simulink model "TechnoEconomicMicrogrid"  (R2025a)
settings: Solver=VariableStepAuto  StartTime=0.0  StopTime=tPeriod-1  FixedStep=sampleTime  RelTol=1e-3
PostLoadFcn:
  | TechnoEconomicAnalysisInput
undefined symbols (not defined in the file): batteryProfile, batteryStorage, DiscIntNeverNeededParam, EMS, generatorProfile, generatorSet, line, loadForecast, mainGrid, optimizationInterval, optimizationMode, solarForecast, solarPV, windFarm, windForecast, windPowerEst
libraries: ee_lib x11, fl_lib x9, simulink x5, eeGeneralControl x4, nesl_utility x3, simulink_extras x1
(part 1 of 2)
CloseFcn:
  | figure1 = findobj('Type', 'figure', 'Name','Power Flow in Microgrid');
  | figure2 = findobj('Type', 'figure', 'Name','plot_PowerFlow');
  | figure3 = findobj('Type', 'figure', 'Name','plot_costComparison');
  | figure4 = findobj('Type', 'figure', 'Name','plot_totalCost');
  | figure5 = findobj('Type', 'figure', 'Name','plot_powerInRange');
  | 
  | if ~isempty(figure1)
  |     close(figure1);
  | end
  | if ~isempty(figure2)
  |     close(figure2);
  | end
  | if ~isempty(figure3)
  |     close(figure3);
  | end
  | if ~isempty(figure4)
  |     close(figure4);
  | end
  | if ~isempty(figure5)
  |     close(figure5);
  | end
  | clear figure1 figure2 figure3 figure4 figure5
  | if bdIsLoaded('SolarMPPTTestHarness')
  |     try
  |         close_system('SolarMPPTTestHarness');
  |     catch
  |     end
  | end
  | if bdIsLoaded('WindMPPTTestHarness')
  |       try
  |         close_system('WindMPPTTestHarness');
  |         catch
  |       end
  | end
settings Model: SimulationMode=accelerator  Creator=skota  LastModifiedBy=skota
settings DataIOCC: SaveOutput=off  DSMLogging=off  SaveTime=off  OutputSaveName=logsout
settings DebuggingCC: SFUnusedDataAndEventsDiag=none
settings ModelReferenceCC: PropagateVarSize=During execution

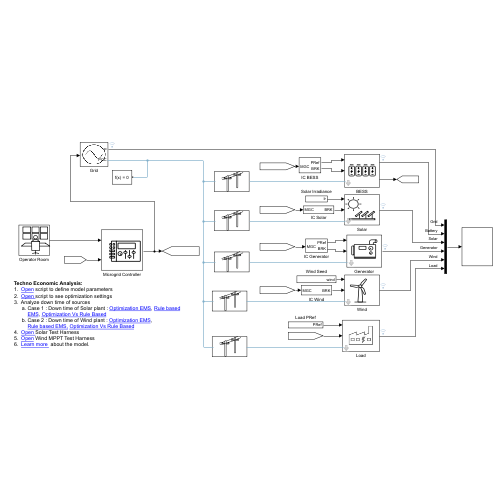
[thumbnail: Simulink's stored preview of the top-level diagram]
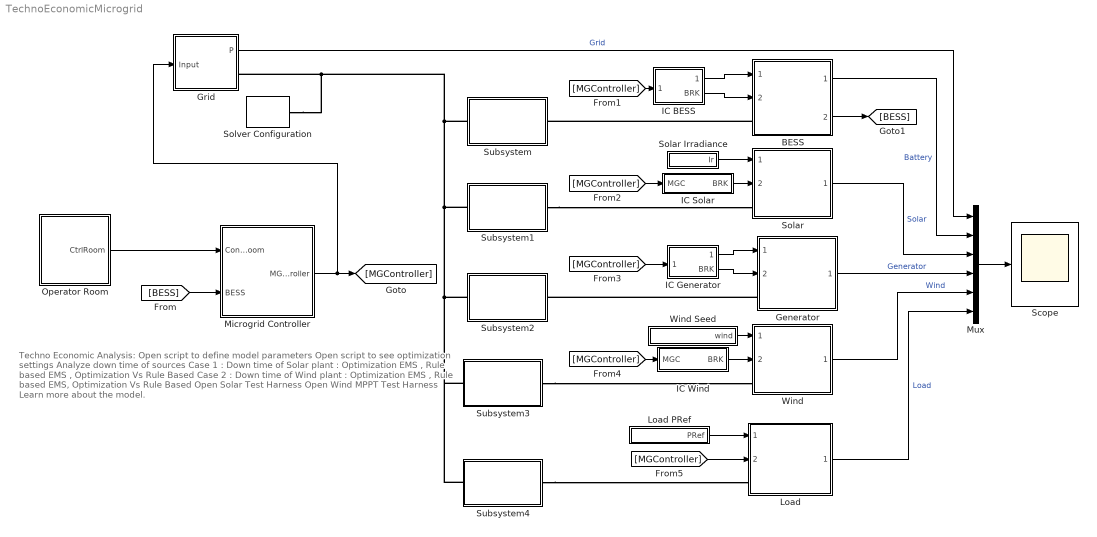
== system TechnoEconomicMicrogrid ==
  note: Techno Economic Analysis:
      | Open script to define model parameters
      | Open script to see optimization settings
      | Analyze down time of sources
      | Case 1 : Down time of Solar plant : Optimization EMS , Rule based EMS , Optimization Vs Rule Based
      | Case 2 : Down time of Wind plant : Optimization EMS ,
      | Rule based EMS, Optimization Vs Rule Based
      | Open Solar Test Harness
      | Open Wind MPPT Test Harness
      | Learn more about the model.
  BESS : Subsystem  ReferencedSubsystem=Battery  minSOC=batteryStorage.minSOC  maxSOC=batteryStorage.maxSOC  energyRating=batteryStorage.energyRating  capacityRating=batteryStorage.capacityRating  nominalVoltage=batteryStorage.nominalVoltage  frequency=systemFrequency  windingRatio=batteryStorage.windingRatio
  Generator : Subsystem  ReferencedSubsystem=Generator  genRating=generatorSet.rating  ratedVoltage=690%generatorSet.voltage  ratedFrequency=systemFrequency  polePairs=generatorSet.polePairs  windingRatio=generatorSet.transformerRatio
  Grid : Subsystem
      settings: PortSchema="{\"entries\":[{\"content\":{\"sides\":[{\"content\":{},\"type\":\"ConnectorPlacement.EquallySpacedRectSide\",\"uuid\":\"0399238b-9a5e-45cc-8714-91426baf51ba\"},{\"content\":{\"side\":\"RIGHT\"},\"type\":\"ConnectorPlacement.EquallySpacedRectSide\",\"uuid\":\"f3b9b3de-730a-435e-bd02-72046c7f84f4\"},{\"content\":{\"connectorIds\":[\"In1\"],\"side\":\"TOP\"},\"type\":\"ConnectorPlacement.EquallySpacedRectSide\",\"uuid\":\"aa72cc88-43a3-4304-9895-61739a7354ea\"},{\"content\":{\"connectorIds\":[\"Out1\",\"RConn1\"],\"side\":\"BOTTOM\"},\"type\":\"ConnectorPlacement.EquallySpacedRectSide\",\"uuid\":\"4abd50ca-018b-43d1-adba-697df11ba2b3\"}]},\"type\":\"ConnectorPlacement.EquallySpacedConnector\",\"uuid\":\"8478d8ff-3240-4ebb-965c-af7f48cfdc7b\"}],\"packageUris\":[\"http://schema.mathworks.com/mf0/Connector/R2020b\"],\"version\":\"1.0\"}"
      mask Display: image('Maingrid.svg');
  IC BESS : Subsystem
  IC Generator : Subsystem
  IC Solar : Subsystem
  IC Wind : Subsystem
  Load : Subsystem  ReferencedSubsystem=Load  windingRatio=loadParam.transformerRatio
  Load PRef : Subsystem
  Microgrid Controller : Subsystem
  Mux : Mux  Inputs=6
  Operator Room : Subsystem
  Scope : Scope
      settings: ActiveDisplayYMinimum=-294.67014  ActiveDisplayYMaximum=1651.08845
  Solar : Subsystem  ReferencedSubsystem=Solar  maxSolarIrradiance=solarPV.maxIrradiance  solarRating=solarPV.rating  ratedVoltage=solarPV.voltage  Voc=solarPV.Voc  panelOutput=solarPV.panelOutput  frequency=systemFrequency  windingRatio=solarPV.transformerRatio  MPPTVoltage=solarMPPT.vMPP  MPPTIrradiance=solarMPPT.irradiance
  Solar Irradiance : Subsystem
  Solver Configuration : nesl_utility/Solver Configuration  PhysicalDomain=network_engine_domain  SubClassName=solver  LeftPortType=input  RightPortType=generic  Tones=[]  Harmonics=[]  SimulateNoise=off  Profile=off  UseLocalSampling=off  EnableSwitchedLinearOptims=on  FrequencyDomain=off  UseCCode=off  RelTol=0.001  AbsTol=0.001  MinStep=1e-09  ToWorkspace=off  RevertToSquareIcSolve=off  NumHomotopyIterations=100  PhasorMode=off  PhasorModeNumHarmonics=1  ConsistencySolver=NEWTON_XTOL_AFTER_FTOL  IndexReductionMethod=DerivativeReplacement  DoDC=off  ResidualTolerance=1e-09  ConsistencyTolSource=GLOBAL  ConsistencyAbsTol=0.001  ConsistencyRelTol=0.001  ConsistencyTolFactor=1  UseLocalSolver=on  LocalSolverChoice=NE_BACKWARD_EULER_ADVANCER  ResolveIndetEquations=on  FunctionEvalNumThread=1  LocalSolverSampleTime=sampleTime  DoFixedCost=on  MaxNonlinIter=3  MaxModeIter=2  ComputeImpulses=off  ImpulseIterations=2  LinearAlgebra=Sparse  LinearAlgebraNumThread=0  EquationFormulation=NE_FREQUENCY_TIME_EF  DelaysMemoryBudget=1024  AutomaticFiltering=on  FilteringTimeConstant=0.001  PartitionStorageMethod=AS_NEEDED  PartitionMemoryBudget=1024  PartitionMethod=ROBUST  MultibodyUseLocalSolver=off  MultibodyLocalSolverChoice=ODE1  MultibodyLocalSolverSampleTime=0.001
  Subsystem : Subsystem
  Subsystem1 : Subsystem
  Subsystem2 : Subsystem
  Subsystem3 : Subsystem
  Subsystem4 : Subsystem
  Wind : Subsystem  ReferencedSubsystem=Wind  windRating=windFarm.rating  maxWindSpeed=windFarm.maxWindSpeed  turbineOutput=windFarm.turbineOutput  frequency=systemFrequency  windingRatio=windFarm.transformerRatio  rotorSpeed=windMPPT.rotorSpeed  windSpeed=windMPPT.windSpeed
  Wind Seed : Subsystem
  wires:
  Grid/1(P) -> Mux/1  "Grid"
  BESS/1 -> Mux/2  "Battery"
  Solar/1 -> Mux/3  "Solar"
  Generator/1 -> Mux/4  "Generator"
  Wind/1 -> Mux/5  "Wind"
  Load/1 -> Mux/6  "Load"
  Operator Room/1(CtrlRoom) -> Microgrid Controller/1(Control Room)
  Microgrid Controller/1(MGController) -> Grid/1(Input), [MGController]
  [BESS] -> Microgrid Controller/2(BESS)
  [MGController] -> IC Wind/1(MGC)
  [MGController] -> Load/2
  Mux/1 -> Scope/1
  BESS/2 -> [BESS]
  [MGController] -> IC BESS/1(MGC)
  IC BESS/2(BRK) -> BESS/2
  IC BESS/1(PRef) -> BESS/1
  [MGController] -> IC Solar/1(MGC)
  IC Solar/1(BRK) -> Solar/2
  IC Wind/1(BRK) -> Wind/2
  Solar Irradiance/1(Ir) -> Solar/1
  IC Generator/1(PRef) -> Generator/1
  Wind Seed/1(wind) -> Wind/1
  Load PRef/1(PRef) -> Load/1
  [MGController] -> IC Generator/1(MGC)
  IC Generator/2(BRK) -> Generator/2
  connections:
  Subsystem4/LConn1 -- Subsystem3/LConn1 -- Subsystem1/LConn1 -- Subsystem/LConn1 -- Solver Configuration/RConn1 -- Grid/RConn1 -- Subsystem2/LConn1
  BESS/LConn1 -- Subsystem/RConn1
  Subsystem1/RConn1 -- Solar/LConn1
  Generator/LConn1 -- Subsystem2/RConn1
  Subsystem3/RConn1 -- Wind/LConn1
  Subsystem4/RConn1 -- Load/LConn1

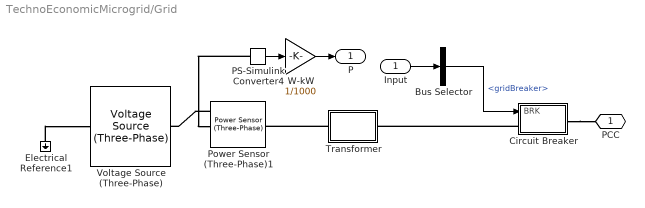
== system TechnoEconomicMicrogrid/Grid ==
  Input : Inport
  Bus Selector : BusSelector  OutputSignals=BrkControl.gridBreaker
  Circuit Breaker : Subsystem
  Electrical Reference1 : fl_lib/Electrical/Electrical Elements/Electrical Reference
  PS-Simulink Converter4 : nesl_utility/PS-Simulink Converter  PhysicalDomain=network_engine_domain  SubClassName=ps_output  LeftPortType=input  RightPortType=output  PseudoPeriodic=off  Frequencies=[]  VectorFormat=inherit  Unit=inherit  AffineConversion=off
  Power Sensor (Three-Phase)1 : ee_lib/Sensors & Transducers/Power Sensor (Three-Phase)  load_type=ee.enum.passive.type_balanced.balanced  f0=60 Hz  config=ee.enum.with_neutral.no  rho=1
      settings: InternalSimscapePortConfiguration="{\"Bottom\":[],\"Left\":[{\"id\":\"N1\",\"label\":\"~1\",\"type\":\"foundation.electrical.three_phase\"}],\"Right\":[{\"id\":\"N2\",\"label\":\"~2\",\"type\":\"foundation.electrical.three_phase\"}],\"Top\":[{\"id\":\"Pm\",\"label\":\"P\",\"type\":\"output\"},{\"id\":\"Qm\",\"label\":\"Q\",\"type\":\"output\"}]}"
  Transformer : Subsystem  mask{windingRatio=mainGrid.transformerRatio}
      mask prompts: windingRatio "Winding ratio"
      mask DialogControl Container4 Prompt: General
  Voltage Source (Three-Phase) : ee_lib/Sources/Voltage Source (Three-Phase)  vline_rms=mainGrid.voltage V  shift=0 deg  freq=systemFrequency Hz  impedance_option=0  SShortCircuit=1e6 A*V  XR=15  R=0.01 Ohm  L=3.97e-4 H  harmonic_option=0  harmonic_orders=[5, 7, 11, 13]  harmonic_ratios=[.1, .1, .1, .1]  G_parasitic=0 1/Ohm  I_specify=off  I_priority=None  I=[0, 0, 0] A  I_nominal_specify=off  I_nominal_value=1  I_nominal_unit=A
  W-kW : Gain  Gain=1/1000
  PCC : PMIOPort  Side=Right
  P : Outport
  wires:
  PS-Simulink Converter4/1 -> W-kW/1
  Bus Selector/1 -> Circuit Breaker/1(BRK)  "<gridBreaker>"
  Input/1 -> Bus Selector/1
  W-kW/1 -> P/1
  connections:
  Power Sensor (Three-Phase)1/LConn1 -- Voltage Source (Three-Phase)/RConn1
  Electrical Reference1/LConn1 -- Voltage Source (Three-Phase)/LConn1
  PS-Simulink Converter4/LConn1 -- Power Sensor (Three-Phase)1/LConn2
  Circuit Breaker/LConn1 -- Transformer/RConn1
  Circuit Breaker/RConn1 -- PCC/RConn1
  Transformer/LConn1 -- Power Sensor (Three-Phase)1/RConn1

== system TechnoEconomicMicrogrid/IC BESS ==
  Bus Element In : Inport  PortName=MGC  Element=bessPRef
  BusElementIn : Inport  PortName=MGC  Element=BrkControl.batteryBreaker
  Delay : Delay  InitialCondition=0.1
  PRef : Outport
  BRK : Outport  Port=2
  wires:
  BusElementIn/1 -> BRK/1
  Bus Element In/1 -> Delay/1
  Delay/1 -> PRef/1

== system TechnoEconomicMicrogrid/IC Generator ==
  BusElementIn : Inport  PortName=MGC  Element=BrkControl.downTime.flag
  BusElementIn3 : Inport  PortName=MGC  Element=BrkControl.generatorBreaker
  BusElementIn1 : Inport  PortName=MGC  Element=genPRef
  From Workspace1 : FromWorkspace  VariableName=generatorProfile(1:nSamples,1:2)
  Switch : Switch  Criteria=u2 > Threshold  SaturateOnIntegerOverflow=off  InputSameDT=off
  PRef : Outport
  BRK : Outport  Port=2
  wires:
  BusElementIn/1 -> Switch/2
  BusElementIn1/1 -> Switch/1
  From Workspace1/1 -> Switch/3
  Switch/1 -> PRef/1
  BusElementIn3/1 -> BRK/1

== system TechnoEconomicMicrogrid/IC Solar ==
  MGC : Inport
  AND : Logic  Operator=OR  AllPortsSameDT=off  OutDataTypeStr=boolean
  Bus Selector : BusSelector  OutputSignals=BrkControl.solarBreaker,BrkControl.downTime.flag
  Compare To Constant : simulink/Logic and Bit Operations/Compare To Constant  relop=>  const=1  OutDataTypeStr=boolean
  BRK : Outport
  wires:
  MGC/1 -> Bus Selector/1
  Compare To Constant/1 -> AND/2
  Bus Selector/2 -> Compare To Constant/1  "<flag>"
  Bus Selector/1 -> AND/1  "<solarBreaker>"
  AND/1 -> BRK/1

== system TechnoEconomicMicrogrid/IC Wind ==
  BusElementIn : Inport  PortName=MGC  Element=BrkControl.downTime.wind
  BusElementIn1 : Inport  PortName=MGC  Element=BrkControl.windBreaker
  Mux : Mux  Inputs=2
  BRK : Outport
  wires:
  BusElementIn/1 -> Mux/1
  BusElementIn1/1 -> Mux/2
  Mux/1 -> BRK/1

== system TechnoEconomicMicrogrid/Load PRef ==
  Delay : Delay  DelayLength=1
  From Workspace2 : FromWorkspace  VariableName=loadForecast(1:nSamples,1:2)
  PRef : Outport
  wires:
  From Workspace2/1 -> Delay/1
  Delay/1 -> PRef/1

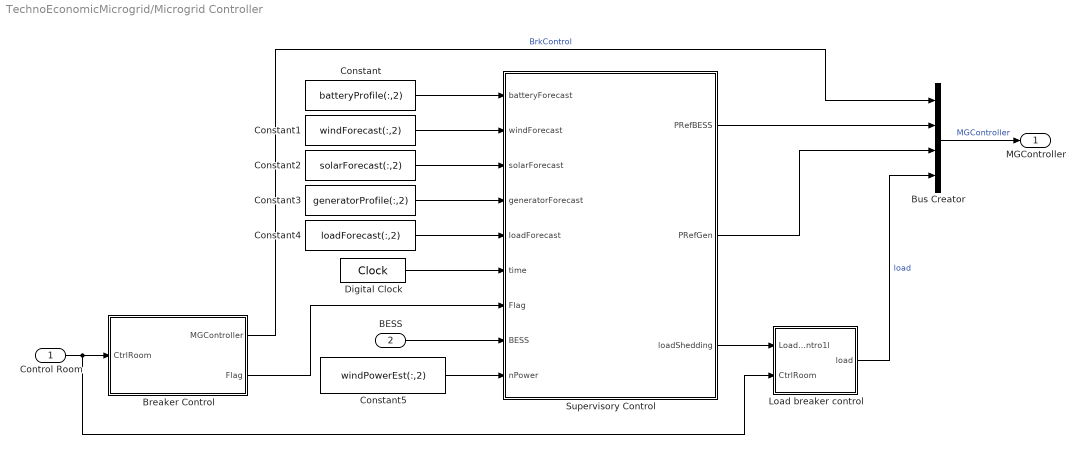
== system TechnoEconomicMicrogrid/Microgrid Controller ==
  Control Room : Inport
  BESS : Inport  Port=2
  Breaker Control : Subsystem
  Bus Creator : BusCreator  Inputs=4
  Constant : Constant  Value=batteryProfile(:,2)
  Constant1 : Constant  Value=windForecast(:,2)
  Constant2 : Constant  Value=solarForecast(:,2)
  Constant3 : Constant  Value=generatorProfile(:,2)
  Constant4 : Constant  Value=loadForecast(:,2)
  Constant5 : Constant  Value=windPowerEst(:,2)
  Digital Clock : DigitalClock
  Load breaker control : Subsystem
  Supervisory Control : Subsystem  TreatAsAtomicUnit=on
  MGController : Outport
  wires:
  Constant4/1 -> Supervisory Control/5(loadForecast)
  Digital Clock/1 -> Supervisory Control/6(time)
  Constant2/1 -> Supervisory Control/3(solarForecast)
  Constant/1 -> Supervisory Control/1(batteryForecast)
  Constant3/1 -> Supervisory Control/4(generatorForecast)
  Constant1/1 -> Supervisory Control/2(windForecast)
  Breaker Control/1(MGController) -> Bus Creator/1  "BrkControl"
  Control Room/1 -> Load breaker control/2(CtrlRoom), Breaker Control/1(CtrlRoom)
  Bus Creator/1 -> MGController/1  "MGController"
  Supervisory Control/1(PRefBESS) -> Bus Creator/2
  Breaker Control/2(Flag) -> Supervisory Control/7(Flag)
  Supervisory Control/3(loadShedding) -> Load breaker control/1(Load Contro1l)
  Load breaker control/1(load) -> Bus Creator/4  "load"
  Supervisory Control/2(PRefGen) -> Bus Creator/3
  BESS/1 -> Supervisory Control/8(BESS)
  Constant5/1 -> Supervisory Control/9(nPower)

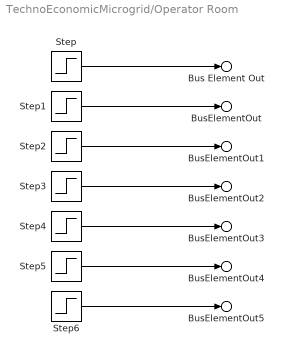
== system TechnoEconomicMicrogrid/Operator Room ==
  Step : Step  Time=solarPV.breakerControl  SampleTime=0
  Step1 : Step  Time=windFarm.breakerControl  SampleTime=0
  Step2 : Step  Time=batteryStorage.breakerControl  SampleTime=0
  Step3 : Step  Time=generatorSet.breakerControl  SampleTime=0
  Step4 : Step  Time=mainGrid.breakerControl  SampleTime=0
  Step5 : Step  Time=mainGrid.breakerControl  SampleTime=0
  Step6 : Step  Time=mainGrid.breakerControl  SampleTime=0
  Bus Element Out : Outport  PortName=CtrlRoom  Element=solarBreaker
  BusElementOut : Outport  PortName=CtrlRoom  Element=windBreaker
  BusElementOut1 : Outport  PortName=CtrlRoom  Element=batteryBreaker
  BusElementOut2 : Outport  PortName=CtrlRoom  Element=generatorBreaker
  BusElementOut3 : Outport  PortName=CtrlRoom  Element=PCCbreaker
  BusElementOut4 : Outport  PortName=CtrlRoom  Element=load1Breaker
  BusElementOut5 : Outport  PortName=CtrlRoom  Element=load2Breaker
  wires:
  Step/1 -> Bus Element Out/1
  Step1/1 -> BusElementOut/1
  Step2/1 -> BusElementOut1/1
  Step3/1 -> BusElementOut2/1
  Step4/1 -> BusElementOut3/1
  Step5/1 -> BusElementOut4/1
  Step6/1 -> BusElementOut5/1

== system TechnoEconomicMicrogrid/Solar Irradiance ==
  Delay : Delay  DelayLength=1
  From Workspace : FromWorkspace  VariableName=solarForecast(1:nSamples,1:2)
  Ir : Outport
  wires:
  From Workspace/1 -> Delay/1
  Delay/1 -> Ir/1

== system TechnoEconomicMicrogrid/Subsystem ==
  RLC (Three-Phase) : ee_lib/Passive/RLC Assemblies/RLC (Three-Phase)  port_option=ee.enum.threePhasePort.composite  component_structure=ee.enum.rlc.structure.R  R=line.resistance Ohm  L=1e-3 H  C=1e-4 F  R_parasitic=0 Ohm  G_parasitic=0 1/Ohm  IL_specify=off  IL_priority=High  IL=[0, 0, 0] A  IL_nominal_specify=off  IL_nominal_value=1  IL_nominal_unit=A  VC_specify=off  VC_priority=High  VC=[0, 0, 0] V  VC_nominal_specify=off  VC_nominal_value=1  VC_nominal_unit=V
      settings: InternalSimscapePortConfiguration="{\"Bottom\":[],\"Left\":[{\"id\":\"N1\",\"label\":\"~1\",\"type\":\"foundation.electrical.three_phase\"}],\"Right\":[{\"id\":\"N2\",\"label\":\"~2\",\"type\":\"foundation.electrical.three_phase\"}],\"Top\":[]}"
  Conn1 : PMIOPort  Side=Left
  Conn2 : PMIOPort  Port=2  Side=Right
  connections:
  RLC (Three-Phase)/LConn1 -- Conn1/RConn1
  RLC (Three-Phase)/RConn1 -- Conn2/RConn1

== system TechnoEconomicMicrogrid/Subsystem1 ==
  RLC (Three-Phase) : ee_lib/Passive/RLC Assemblies/RLC (Three-Phase)  port_option=ee.enum.threePhasePort.composite  component_structure=ee.enum.rlc.structure.R  R=line.resistance Ohm  L=1e-3 H  C=1e-4 F  R_parasitic=0 Ohm  G_parasitic=0 1/Ohm  IL_specify=off  IL_priority=High  IL=[0, 0, 0] A  IL_nominal_specify=off  IL_nominal_value=1  IL_nominal_unit=A  VC_specify=off  VC_priority=High  VC=[0, 0, 0] V  VC_nominal_specify=off  VC_nominal_value=1  VC_nominal_unit=V
      settings: InternalSimscapePortConfiguration="{\"Bottom\":[],\"Left\":[{\"id\":\"N1\",\"label\":\"~1\",\"type\":\"foundation.electrical.three_phase\"}],\"Right\":[{\"id\":\"N2\",\"label\":\"~2\",\"type\":\"foundation.electrical.three_phase\"}],\"Top\":[]}"
  Conn1 : PMIOPort  Side=Left
  Conn2 : PMIOPort  Port=2  Side=Right
  connections:
  RLC (Three-Phase)/LConn1 -- Conn1/RConn1
  RLC (Three-Phase)/RConn1 -- Conn2/RConn1

== system TechnoEconomicMicrogrid/Subsystem2 ==
  RLC (Three-Phase) : ee_lib/Passive/RLC Assemblies/RLC (Three-Phase)  port_option=ee.enum.threePhasePort.composite  component_structure=ee.enum.rlc.structure.R  R=line.resistance Ohm  L=1e-3 H  C=1e-4 F  R_parasitic=0 Ohm  G_parasitic=0 1/Ohm  IL_specify=off  IL_priority=High  IL=[0, 0, 0] A  IL_nominal_specify=off  IL_nominal_value=1  IL_nominal_unit=A  VC_specify=off  VC_priority=High  VC=[0, 0, 0] V  VC_nominal_specify=off  VC_nominal_value=1  VC_nominal_unit=V
      settings: InternalSimscapePortConfiguration="{\"Bottom\":[],\"Left\":[{\"id\":\"N1\",\"label\":\"~1\",\"type\":\"foundation.electrical.three_phase\"}],\"Right\":[{\"id\":\"N2\",\"label\":\"~2\",\"type\":\"foundation.electrical.three_phase\"}],\"Top\":[]}"
  Conn1 : PMIOPort  Side=Left
  Conn2 : PMIOPort  Port=2  Side=Right
  connections:
  RLC (Three-Phase)/LConn1 -- Conn1/RConn1
  RLC (Three-Phase)/RConn1 -- Conn2/RConn1

== system TechnoEconomicMicrogrid/Subsystem3 ==
  RLC (Three-Phase) : ee_lib/Passive/RLC Assemblies/RLC (Three-Phase)  port_option=ee.enum.threePhasePort.composite  component_structure=ee.enum.rlc.structure.R  R=line.resistance Ohm  L=1e-3 H  C=1e-4 F  R_parasitic=0 Ohm  G_parasitic=0 1/Ohm  IL_specify=off  IL_priority=High  IL=[0, 0, 0] A  IL_nominal_specify=off  IL_nominal_value=1  IL_nominal_unit=A  VC_specify=off  VC_priority=High  VC=[0, 0, 0] V  VC_nominal_specify=off  VC_nominal_value=1  VC_nominal_unit=V
      settings: InternalSimscapePortConfiguration="{\"Bottom\":[],\"Left\":[{\"id\":\"N1\",\"label\":\"~1\",\"type\":\"foundation.electrical.three_phase\"}],\"Right\":[{\"id\":\"N2\",\"label\":\"~2\",\"type\":\"foundation.electrical.three_phase\"}],\"Top\":[]}"
  Conn1 : PMIOPort  Side=Left
  Conn2 : PMIOPort  Port=2  Side=Right
  connections:
  RLC (Three-Phase)/LConn1 -- Conn1/RConn1
  RLC (Three-Phase)/RConn1 -- Conn2/RConn1

== system TechnoEconomicMicrogrid/Subsystem4 ==
  RLC (Three-Phase) : ee_lib/Passive/RLC Assemblies/RLC (Three-Phase)  port_option=ee.enum.threePhasePort.composite  component_structure=ee.enum.rlc.structure.R  R=line.resistance Ohm  L=1e-3 H  C=1e-4 F  R_parasitic=0 Ohm  G_parasitic=0 1/Ohm  IL_specify=off  IL_priority=High  IL=[0, 0, 0] A  IL_nominal_specify=off  IL_nominal_value=1  IL_nominal_unit=A  VC_specify=off  VC_priority=High  VC=[0, 0, 0] V  VC_nominal_specify=off  VC_nominal_value=1  VC_nominal_unit=V
      settings: InternalSimscapePortConfiguration="{\"Bottom\":[],\"Left\":[{\"id\":\"N1\",\"label\":\"~1\",\"type\":\"foundation.electrical.three_phase\"}],\"Right\":[{\"id\":\"N2\",\"label\":\"~2\",\"type\":\"foundation.electrical.three_phase\"}],\"Top\":[]}"
  Conn1 : PMIOPort  Side=Left
  Conn2 : PMIOPort  Port=2  Side=Right
  connections:
  RLC (Three-Phase)/LConn1 -- Conn1/RConn1
  RLC (Three-Phase)/RConn1 -- Conn2/RConn1

== system TechnoEconomicMicrogrid/Wind Seed ==
  From Workspace4 : FromWorkspace  VariableName=windForecast(1:nSamples,1:2)
  wind : Outport
  wires:
  From Workspace4/1 -> wind/1

== system TechnoEconomicMicrogrid/Grid/Circuit Breaker ==
  BRK : Inport
  Data Type Conversion : DataTypeConversion  OutDataTypeStr=double  SaturateOnIntegerOverflow=off  RndMeth=Floor
  Open Resistance : Gain  Gain=1e5
  Phase Splitter : ee_lib/Connectors & References/Phase Splitter
  Phase Splitter1 : ee_lib/Connectors & References/Phase Splitter
  Simulink-PS Converter : nesl_utility/Simulink-PS Converter  PhysicalDomain=network_engine_domain  SubClassName=ps_input  LeftPortType=input  RightPortType=output  PseudoPeriodic=off  Frequencies=[]  NoiseDistribution=none  NoiseParameters=[]  Unit=1  AffineConversion=off  FilteringAndDerivatives=provide  SimscapeFilterOrder=1  InputFilterTimeConstant=0.001  UdotUserProvided=0
  Variable Resistor : fl_lib/Electrical/Electrical Elements/Variable Resistor  Rmin=1e-4 Ohm  thermalEnable=false  thermal_mass=1 J/K  i_specify=off  i_priority=None  i=0 A  i_nominal_specify=off  i_nominal_value=1  i_nominal_unit=A  v_specify=off  v_priority=None  v=0 V  v_nominal_specify=off  v_nominal_value=1  v_nominal_unit=V  T_specify=off  T_priority=None  T=300 K  T_nominal_specify=off  T_nominal_value=1  T_nominal_unit=K
  Variable Resistor1 : fl_lib/Electrical/Electrical Elements/Variable Resistor  Rmin=1e-4 Ohm  thermalEnable=false  thermal_mass=1 J/K  i_specify=off  i_priority=None  i=0 A  i_nominal_specify=off  i_nominal_value=1  i_nominal_unit=A  v_specify=off  v_priority=None  v=0 V  v_nominal_specify=off  v_nominal_value=1  v_nominal_unit=V  T_specify=off  T_priority=None  T=300 K  T_nominal_specify=off  T_nominal_value=1  T_nominal_unit=K
  Variable Resistor2 : fl_lib/Electrical/Electrical Elements/Variable Resistor  Rmin=1e-4 Ohm  thermalEnable=false  thermal_mass=1 J/K  i_specify=off  i_priority=None  i=0 A  i_nominal_specify=off  i_nominal_value=1  i_nominal_unit=A  v_specify=off  v_priority=None  v=0 V  v_nominal_specify=off  v_nominal_value=1  v_nominal_unit=V  T_specify=off  T_priority=None  T=300 K  T_nominal_specify=off  T_nominal_value=1  T_nominal_unit=K
  In : PMIOPort  Side=Left
  ~ : PMIOPort  Port=2  Side=Right
  wires:
  Data Type Conversion/1 -> Open Resistance/1
  BRK/1 -> Data Type Conversion/1
  Open Resistance/1 -> Simulink-PS Converter/1
  connections:
  Phase Splitter1/RConn2 -- Variable Resistor1/RConn1
  Variable Resistor1/LConn2 -- Phase Splitter/RConn2
  Phase Splitter1/RConn3 -- Variable Resistor2/RConn1
  Phase Splitter/RConn1 -- Variable Resistor/LConn2
  Variable Resistor2/LConn2 -- Phase Splitter/RConn3
  Phase Splitter1/RConn1 -- Variable Resistor/RConn1
  Phase Splitter1/LConn1 -- ~/RConn1
  Variable Resistor/LConn1 -- Simulink-PS Converter/RConn1 -- Variable Resistor2/LConn1 -- Variable Resistor1/LConn1
  Phase Splitter/LConn1 -- In/RConn1

== system TechnoEconomicMicrogrid/Grid/Transformer ==
  Electrical Reference : fl_lib/Electrical/Electrical Elements/Electrical Reference
  Electrical Reference1 : fl_lib/Electrical/Electrical Elements/Electrical Reference
  Ideal Transformer : fl_lib/Electrical/Electrical Elements/Ideal Transformer  n=windingRatio  i1_specify=off  i1_priority=None  i1=0 A  i1_nominal_specify=off  i1_nominal_value=1  i1_nominal_unit=A  v1_specify=off  v1_priority=None  v1=0 V  v1_nominal_specify=off  v1_nominal_value=1  v1_nominal_unit=V  i2_specify=off  i2_priority=None  i2=0 A  i2_nominal_specify=off  i2_nominal_value=1  i2_nominal_unit=A  v2_specify=off  v2_priority=None  v2=0 V  v2_nominal_specify=off  v2_nominal_value=1  v2_nominal_unit=V
  Ideal Transformer1 : fl_lib/Electrical/Electrical Elements/Ideal Transformer  n=windingRatio  i1_specify=off  i1_priority=None  i1=0 A  i1_nominal_specify=off  i1_nominal_value=1  i1_nominal_unit=A  v1_specify=off  v1_priority=None  v1=0 V  v1_nominal_specify=off  v1_nominal_value=1  v1_nominal_unit=V  i2_specify=off  i2_priority=None  i2=0 A  i2_nominal_specify=off  i2_nominal_value=1  i2_nominal_unit=A  v2_specify=off  v2_priority=None  v2=0 V  v2_nominal_specify=off  v2_nominal_value=1  v2_nominal_unit=V
  Ideal Transformer2 : fl_lib/Electrical/Electrical Elements/Ideal Transformer  n=windingRatio  i1_specify=off  i1_priority=None  i1=0 A  i1_nominal_specify=off  i1_nominal_value=1  i1_nominal_unit=A  v1_specify=off  v1_priority=None  v1=0 V  v1_nominal_specify=off  v1_nominal_value=1  v1_nominal_unit=V  i2_specify=off  i2_priority=None  i2=0 A  i2_nominal_specify=off  i2_nominal_value=1  i2_nominal_unit=A  v2_specify=off  v2_priority=None  v2=0 V  v2_nominal_specify=off  v2_nominal_value=1  v2_nominal_unit=V
  Phase Splitter : ee_lib/Connectors & References/Phase Splitter
  Phase Splitter1 : ee_lib/Connectors & References/Phase Splitter
  In : PMIOPort  Side=Left
  Out : PMIOPort  Port=2  Side=Right
  connections:
  Ideal Transformer1/RConn1 -- Phase Splitter1/RConn2
  Ideal Transformer2/RConn1 -- Phase Splitter1/RConn3
  Ideal Transformer/RConn1 -- Phase Splitter1/RConn1
  Phase Splitter1/LConn1 -- Out/RConn1
  Phase Splitter/LConn1 -- In/RConn1
  Ideal Transformer2/LConn2 -- Ideal Transformer1/LConn2 -- Electrical Reference/LConn1 -- Ideal Transformer/LConn2
  Phase Splitter/RConn1 -- Ideal Transformer/LConn1
  Phase Splitter/RConn2 -- Ideal Transformer1/LConn1
  Phase Splitter/RConn3 -- Ideal Transformer2/LConn1
  Ideal Transformer2/RConn2 -- Ideal Transformer1/RConn2 -- Electrical Reference1/LConn1 -- Ideal Transformer/RConn2

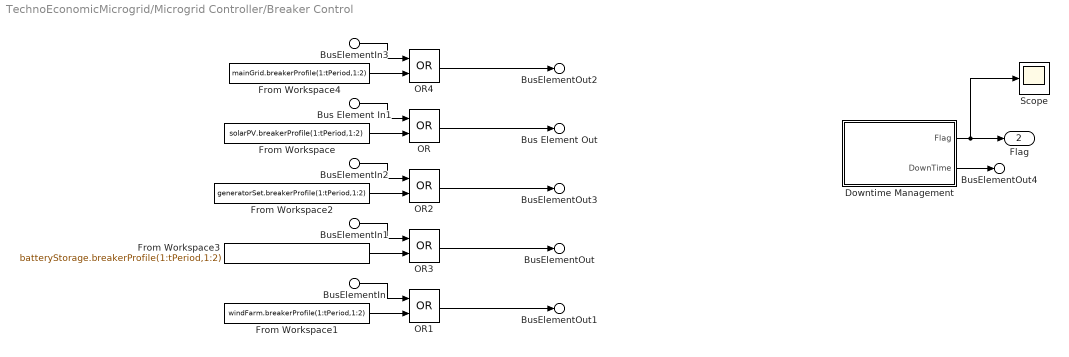
== system TechnoEconomicMicrogrid/Microgrid Controller/Breaker Control ==
  Bus Element In1 : Inport  PortName=CtrlRoom  Element=solarBreaker
  BusElementIn : Inport  PortName=CtrlRoom  Element=windBreaker
  BusElementIn1 : Inport  PortName=CtrlRoom  Element=batteryBreaker
  BusElementIn2 : Inport  PortName=CtrlRoom  Element=generatorBreaker
  BusElementIn3 : Inport  PortName=CtrlRoom  Element=PCCbreaker
  Downtime Management : Subsystem
  From Workspace : FromWorkspace  VariableName=solarPV.breakerProfile(1:tPeriod,1:2)
  From Workspace1 : FromWorkspace  VariableName=windFarm.breakerProfile(1:tPeriod,1:2)
  From Workspace2 : FromWorkspace  VariableName=generatorSet.breakerProfile(1:tPeriod,1:2)
  From Workspace3 : FromWorkspace  VariableName=batteryStorage.breakerProfile(1:tPeriod,1:2)
  From Workspace4 : FromWorkspace  VariableName=mainGrid.breakerProfile(1:tPeriod,1:2)
  OR{,1..4} (5 alike) : Logic  Operator=OR  AllPortsSameDT=off  OutDataTypeStr=boolean
  Scope : Scope
      settings: ActiveDisplayYMinimum=-1  ActiveDisplayYMaximum=1  DataLoggingVariableName=ScopeData17
  Bus Element Out : Outport  PortName=MGController  Element=solarBreaker
  BusElementOut : Outport  PortName=MGController  Element=batteryBreaker
  BusElementOut1 : Outport  PortName=MGController  Element=windBreaker
  BusElementOut2 : Outport  PortName=MGController  Element=gridBreaker
  BusElementOut3 : Outport  PortName=MGController  Element=generatorBreaker
  BusElementOut4 : Outport  PortName=MGController  Element=downTime
  Flag : Outport  Port=2
  wires:
  From Workspace2/1 -> OR2/2
  OR/1 -> Bus Element Out/1
  Bus Element In1/1 -> OR/1
  From Workspace4/1 -> OR4/2
  OR4/1 -> BusElementOut2/1
  From Workspace3/1 -> OR3/2
  BusElementIn1/1 -> OR3/1
  From Workspace/1 -> OR/2
  OR2/1 -> BusElementOut3/1
  OR3/1 -> BusElementOut/1
  BusElementIn/1 -> OR1/1
  From Workspace1/1 -> OR1/2
  BusElementIn3/1 -> OR4/1
  OR1/1 -> BusElementOut1/1
  BusElementIn2/1 -> OR2/1
  Downtime Management/1(Flag) -> Scope/1, Flag/1
  Downtime Management/2(DownTime) -> BusElementOut4/1

== system TechnoEconomicMicrogrid/Microgrid Controller/Load breaker control ==
  Load Contro1l : Inport
  Bus Element In : Inport  Port=2  PortName=CtrlRoom  Element=load1Breaker
  BusElementIn : Inport  Port=2  PortName=CtrlRoom  Element=load2Breaker
  Delay : Delay  DelayLength=1
  OR : Logic  Operator=OR  IconShape=distinctive  AllPortsSameDT=off  OutDataTypeStr=boolean
  Out Bus Element : Outport  PortName=load  Element=brk1
  BusElementOut : Outport  PortName=load  Element=brk2
  wires:
  BusElementIn/1 -> OR/1
  Load Contro1l/1 -> Delay/1
  Bus Element In/1 -> Out Bus Element/1
  OR/1 -> BusElementOut/1
  Delay/1 -> OR/2

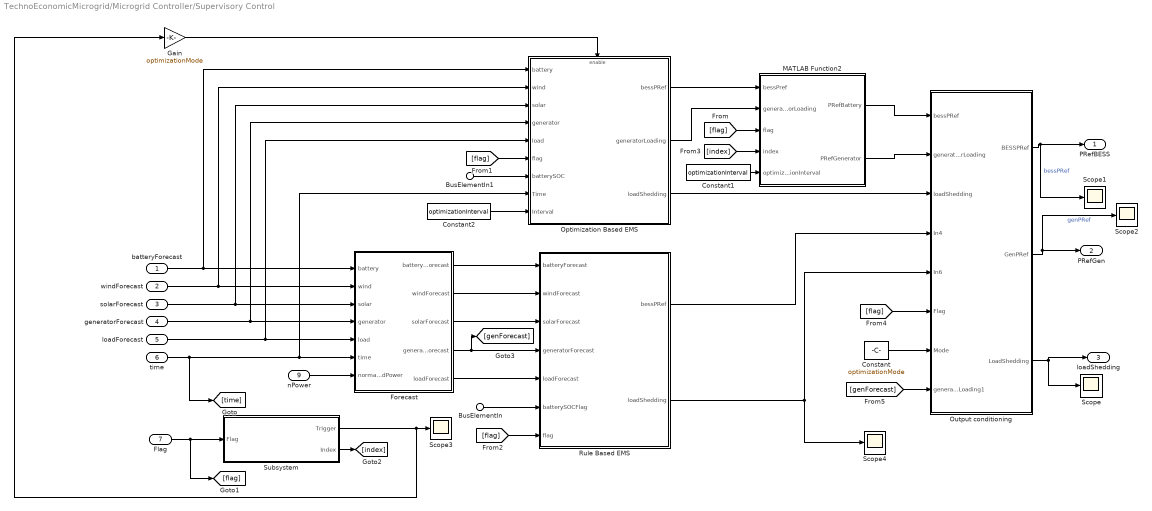
== system TechnoEconomicMicrogrid/Microgrid Controller/Supervisory Control ==
  batteryForecast : Inport
  windForecast : Inport  Port=2
  solarForecast : Inport  Port=3
  generatorForecast : Inport  Port=4
  loadForecast : Inport  Port=5
  time : Inport  Port=6
  Flag : Inport  Port=7
  BusElementIn1 : Inport  Port=8  PortName=BESS  Element=SOC
  BusElementIn : Inport  Port=8  PortName=BESS  Element=SOCFlag
  nPower : Inport  Port=9
  Constant : Constant  Value=optimizationMode
  Constant1 : Constant  Value=optimizationInterval  VectorParams1D=off  SampleTime=-1
  Constant2 : Constant  Value=optimizationInterval  VectorParams1D=off  SampleTime=-1
  Forecast : MATLAB Function  TreatAsAtomicUnit=on
  Gain : Gain  Gain=optimizationMode
  MATLAB Function2 : MATLAB Function  TreatAsAtomicUnit=on
  Optimization Based EMS : Subsystem
  Output conditioning : Subsystem
  Rule Based EMS : Stateflow chart  TreatAsAtomicUnit=on  mask{batteryMaxPower=EMS.maxBatteryPower, batteryMinSOC=EMS.minBatterySOC, batteryMaxSOC=EMS.maxBatterySOC, gridPowerMax=EMS.maxGridPower, windRating=windFarm.rating, solarRating=solarPV.rating, generatorRating=generatorSet.rating}
      mask prompts: batteryMaxPower "Maximum Battery Power"; batteryMinSOC "Minimum Battery SOC"; batteryMaxSOC "Maximum Battery SOC"; gridPowerMax "Maximum Grid Power"; windRating "Rating"; solarRating "Rating"; generatorRating "Rating"
  Scope{,1..4} (5 alike) : Scope
      Scope settings: ActiveDisplayYMinimum=-0.125  ActiveDisplayYMaximum=1.125  DataLoggingVariableName=ScopeData5
      Scope1 settings: ActiveDisplayYMinimum=-65350.65429  ActiveDisplayYMaximum=36094.11923  DataLoggingVariableName=ScopeData6
      Scope2 settings: ActiveDisplayYMinimum=0.2125  ActiveDisplayYMaximum=1.0875  DataLoggingVariableName=ScopeData7
      Scope3 settings: ActiveDisplayYMinimum=-0.04865  ActiveDisplayYMaximum=1.01271  DataLoggingVariableName=ScopeData9
      Scope4 settings: ActiveDisplayYMinimum=-1  ActiveDisplayYMaximum=1  DataLoggingVariableName=ScopeData9
  Subsystem : Subsystem
  PRefBESS : Outport
  PRefGen : Outport  Port=2
  loadShedding : Outport  Port=3
  wires:
  batteryForecast/1 -> Optimization Based EMS/1(battery), Forecast/1(battery)
  solarForecast/1 -> Optimization Based EMS/3(solar), Forecast/3(solar)
  windForecast/1 -> Optimization Based EMS/2(wind), Forecast/2(wind)
  generatorForecast/1 -> Optimization Based EMS/4(generator), Forecast/4(generator)
  loadForecast/1 -> Optimization Based EMS/5(load), Forecast/5(load)
  time/1 -> [time], Optimization Based EMS/8(Time), Forecast/6(time)
  Forecast/1(batteryForecast) -> Rule Based EMS/1(batteryForecast)
  Forecast/3(solarForecast) -> Rule Based EMS/3(solarForecast)
  Forecast/4(generatorForecast) -> [genForecast], Rule Based EMS/4(generatorForecast)
  Forecast/5(loadForecast) -> Rule Based EMS/5(loadForecast)
  Forecast/2(windForecast) -> Rule Based EMS/2(windForecast)
  BusElementIn/1 -> Rule Based EMS/6(batterySOCFlag)
  BusElementIn1/1 -> Optimization Based EMS/7(batterySOC)
  Optimization Based EMS/3(loadShedding) -> Output conditioning/3(loadShedding)
  Rule Based EMS/1(bessPRef) -> Output conditioning/4(In4)
  Rule Based EMS/2(loadShedding) -> Output conditioning/5(In6), Scope4/1
  Output conditioning/1(BESSPRef) -> PRefBESS/1, Scope1/1  "bessPRef"
  Output conditioning/2(GenPRef) -> Scope2/1, PRefGen/1  "genPRef"
  Output conditioning/3(LoadShedding) -> loadShedding/1, Scope/1
  Flag/1 -> [flag], Subsystem/1(Flag)
  Subsystem/1(Trigger) -> Gain/1, Scope3/1
  Optimization Based EMS/1(bessPRef) -> MATLAB Function2/1(bessPref)
  Optimization Based EMS/2(generatorLoading) -> MATLAB Function2/2(generatorLoading)
  MATLAB Function2/1(PRefBattery) -> Output conditioning/1(bessPRef)
  MATLAB Function2/2(PRefGenerator) -> Output conditioning/2(generatorLoading)
  [flag] -> Optimization Based EMS/6(flag)
  [flag] -> Rule Based EMS/7(flag)
  [flag] -> Output conditioning/6(Flag)
  Subsystem/2(Index) -> [index]
  [flag] -> MATLAB Function2/3(flag)
  [index] -> MATLAB Function2/4(index)
  Constant/1 -> Output conditioning/7(Mode)
  Gain/1 -> Optimization Based EMS/Enable
  [genForecast] -> Output conditioning/8(generatorLoading1)
  nPower/1 -> Forecast/7(normalizedWindPower)
  Constant1/1 -> MATLAB Function2/5(optimizationInterval)
  Constant2/1 -> Optimization Based EMS/9(Interval)

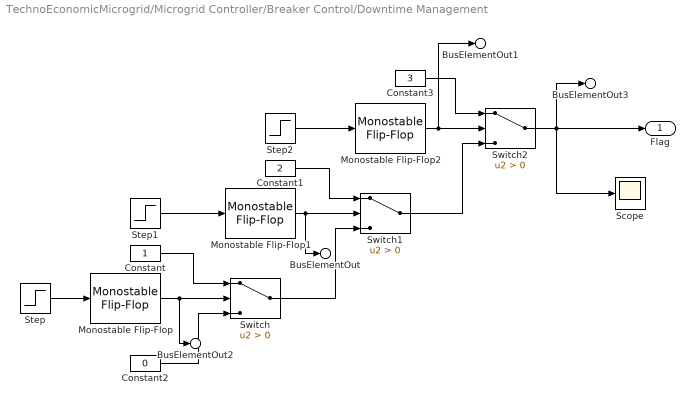
== system TechnoEconomicMicrogrid/Microgrid Controller/Breaker Control/Downtime Management ==
  Constant : Constant
  Constant1 : Constant  Value=2
  Constant2 : Constant  Value=0
  Constant3 : Constant  Value=3
  Monostable Flip-Flop : eeGeneralControl/Monostable Flip-Flop  VariantControl=Variant1  LabelModeActiveChoice=Discrete  ChangeType=Rising edge  x0=0  Td=windFarm.downTimeDuration  Ts=1
      settings: LibrarySourceBlock=ee_sl_lib/General Control/Monostable Flip-Flop
  Monostable Flip-Flop1 : eeGeneralControl/Monostable Flip-Flop  VariantControl=Variant1  LabelModeActiveChoice=Discrete  ChangeType=Rising edge  x0=0  Td=solarPV.downTimeDuration  Ts=1
      settings: LibrarySourceBlock=ee_sl_lib/General Control/Monostable Flip-Flop
  Monostable Flip-Flop2 : eeGeneralControl/Monostable Flip-Flop  VariantControl=Variant1  LabelModeActiveChoice=Discrete  ChangeType=Rising edge  x0=0  Td=generatorSet.downTimeDuration  Ts=1
      settings: LibrarySourceBlock=ee_sl_lib/General Control/Monostable Flip-Flop
  Scope : Scope
      settings: ActiveDisplayYMinimum=-0.25  ActiveDisplayYMaximum=2.25  DataLoggingVariableName=ScopeData19
  Step : Step  Time=windFarm.downTime  SampleTime=0
  Step1 : Step  Time=solarPV.downTime  SampleTime=0
  Step2 : Step  Time=generatorSet.downTime  SampleTime=0
  Switch : Switch  Criteria=u2 > Threshold  SaturateOnIntegerOverflow=off  InputSameDT=off
  Switch1 : Switch  Criteria=u2 > Threshold  SaturateOnIntegerOverflow=off  InputSameDT=off
  Switch2 : Switch  Criteria=u2 > Threshold  SaturateOnIntegerOverflow=off  InputSameDT=off
  Flag : Outport
  BusElementOut2 : Outport  Port=2  PortName=DownTime  Element=wind
  BusElementOut : Outport  Port=2  PortName=DownTime  Element=solar
  BusElementOut1 : Outport  Port=2  PortName=DownTime  Element=generator
  BusElementOut3 : Outport  Port=2  PortName=DownTime  Element=flag
  wires:
  Monostable Flip-Flop/1 -> BusElementOut2/1, Switch/2
  Constant/1 -> Switch/1
  Step/1 -> Monostable Flip-Flop/1
  Step1/1 -> Monostable Flip-Flop1/1
  Monostable Flip-Flop1/1 -> BusElementOut/1, Switch1/2
  Constant1/1 -> Switch1/1
  Constant2/1 -> Switch/3
  Monostable Flip-Flop2/1 -> BusElementOut1/1, Switch2/2
  Step2/1 -> Monostable Flip-Flop2/1
  Switch/1 -> Switch1/3
  Constant3/1 -> Switch2/1
  Switch1/1 -> Switch2/3
  Switch2/1 -> BusElementOut3/1, Scope/1, Flag/1

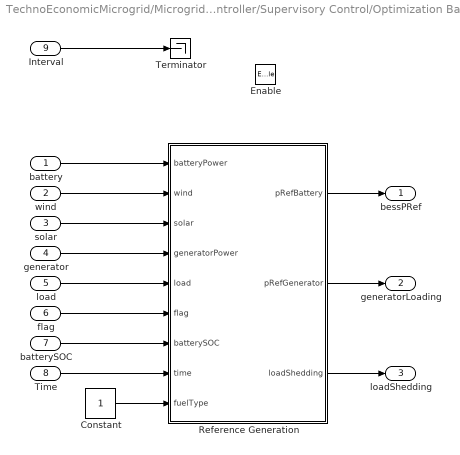
== system TechnoEconomicMicrogrid/Microgrid Controller/Supervisory Control/Optimization Based EMS ==
  battery : Inport
  wind : Inport  Port=2
  solar : Inport  Port=3
  generator : Inport  Port=4
  load : Inport  Port=5
  flag : Inport  Port=6
  batterySOC : Inport  Port=7
  Time : Inport  Port=8
  Interval : Inport  Port=9
  Enable : EnablePort
  Constant : Constant
  Reference Generation : MATLAB Function  TreatAsAtomicUnit=on  mask{generatorRating=generatorSet.rating, solarRating=solarPV.rating, windRating=windFarm.rating, batteryEnergyRating=batteryStorage.energyRating, batteryMaxPower=EMS.maxBatteryPower, gridMaxPower=EMS.maxGridPower, batteryMaxSOC=EMS.maxBatterySOC, batteryMinPower=EMS.minBatteryPower, gridMinPower=EMS.minGridPower, batteryMinSOC=EMS.minBatterySOC, fuelCost=generatorSet.fuelCost, gridCost=mainGrid.cost}
      mask prompts: generatorRating "Generator"; solarRating "Solar"; windRating "Wind"; batteryEnergyRating "Battery Energy"; batteryMaxPower "Battery Power"; gridMaxPower "Grid power"; batteryMaxSOC "Battery SOC"; batteryMinPower "Battery Power"; gridMinPower "Grid Power"; batteryMinSOC "Battery SOC"; fuelCost "Generator Fuel Cost"; gridCost "Grid price"
  Terminator : Terminator
  bessPRef : Outport
  generatorLoading : Outport  Port=2
  loadShedding : Outport  Port=3
  wires:
  solar/1 -> Reference Generation/3(solar)
  batterySOC/1 -> Reference Generation/7(batterySOC)
  wind/1 -> Reference Generation/2(wind)
  flag/1 -> Reference Generation/6(flag)
  Interval/1 -> Terminator/1
  battery/1 -> Reference Generation/1(batteryPower)
  load/1 -> Reference Generation/5(load)
  Time/1 -> Reference Generation/8(time)
  generator/1 -> Reference Generation/4(generatorPower)
  Reference Generation/1(pRefBattery) -> bessPRef/1
  Reference Generation/2(pRefGenerator) -> generatorLoading/1
  Reference Generation/3(loadShedding) -> loadShedding/1
  Constant/1 -> Reference Generation/9(fuelType)

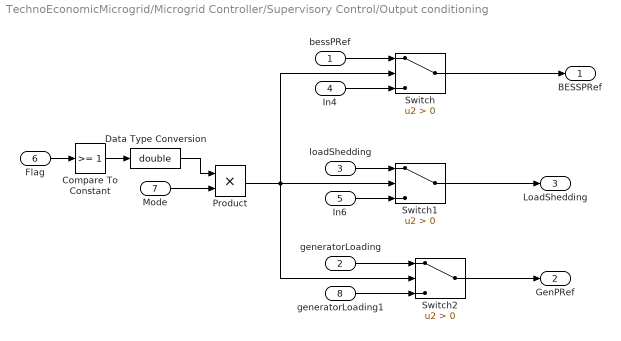
== system TechnoEconomicMicrogrid/Microgrid Controller/Supervisory Control/Output conditioning ==
  bessPRef : Inport
  generatorLoading : Inport  Port=2
  loadShedding : Inport  Port=3
  In4 : Inport  Port=4
  In6 : Inport  Port=5
  Flag : Inport  Port=6
  Mode : Inport  Port=7
  generatorLoading1 : Inport  Port=8
  Compare To Constant : simulink/Logic and Bit Operations/Compare To Constant  relop=>=  const=1  OutDataTypeStr=boolean
  Data Type Conversion : DataTypeConversion  OutDataTypeStr=double  SaturateOnIntegerOverflow=off  RndMeth=Floor
  Product : Product
  Switch : Switch  Criteria=u2 > Threshold  SaturateOnIntegerOverflow=off  InputSameDT=off
  Switch1 : Switch  Criteria=u2 > Threshold  SaturateOnIntegerOverflow=off  InputSameDT=off
  Switch2 : Switch  Criteria=u2 > Threshold  SaturateOnIntegerOverflow=off  InputSameDT=off
  BESSPRef : Outport
  GenPRef : Outport  Port=2
  LoadShedding : Outport  Port=3
  wires:
  bessPRef/1 -> Switch/1
  In4/1 -> Switch/3
  In6/1 -> Switch1/3
  Switch/1 -> BESSPRef/1
  Flag/1 -> Compare To Constant/1
  loadShedding/1 -> Switch1/1
  Switch1/1 -> LoadShedding/1
  Compare To Constant/1 -> Data Type Conversion/1
  Mode/1 -> Product/2
  Data Type Conversion/1 -> Product/1
  Product/1 -> Switch2/2, Switch1/2, Switch/2
  generatorLoading/1 -> Switch2/1
  generatorLoading1/1 -> Switch2/3
  Switch2/1 -> GenPRef/1

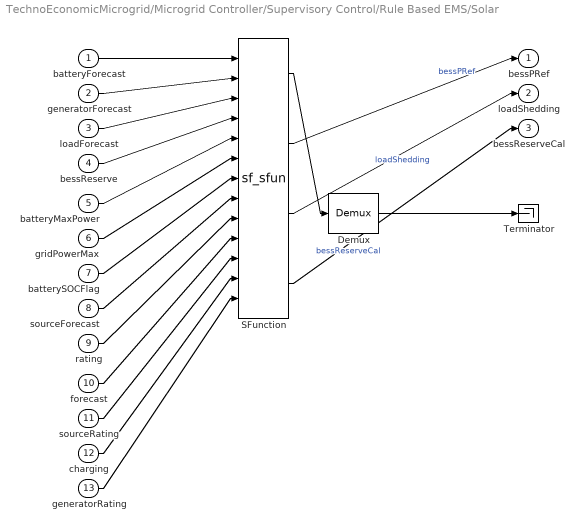
== system TechnoEconomicMicrogrid/Microgrid Controller/Supervisory Control/Rule Based EMS/Solar ==
  batteryForecast : Inport
  generatorForecast : Inport  Port=2
  loadForecast : Inport  Port=3
  bessReserve : Inport  Port=4
  batteryMaxPower : Inport  Port=5
  gridPowerMax : Inport  Port=6
  batterySOCFlag : Inport  Port=7
  sourceForecast : Inport  Port=8
  rating : Inport  Port=9
  forecast : Inport  Port=10
  sourceRating : Inport  Port=11
  charging : Inport  Port=12
  generatorRating : Inport  Port=13
  " Demux " : Demux  Outputs=1
  " SFunction " : S-Function  Tag=Stateflow S-Function 1  FunctionName=sf_sfun  PortCounts=[13 4]  SFunctionDeploymentMode=off  EnableBusSupport=off
  " Terminator " : Terminator
  bessPRef : Outport
  loadShedding : Outport  Port=2
  bessReserveCal : Outport  Port=3
  wires:
  batteryForecast/1 -> " SFunction "/1
  generatorForecast/1 -> " SFunction "/2
  loadForecast/1 -> " SFunction "/3
  bessReserve/1 -> " SFunction "/4
  batteryMaxPower/1 -> " SFunction "/5
  gridPowerMax/1 -> " SFunction "/6
  batterySOCFlag/1 -> " SFunction "/7
  sourceForecast/1 -> " SFunction "/8
  rating/1 -> " SFunction "/9
  forecast/1 -> " SFunction "/10
  sourceRating/1 -> " SFunction "/11
  charging/1 -> " SFunction "/12
  generatorRating/1 -> " SFunction "/13
  " SFunction "/2 -> bessPRef/1  "bessPRef"
  " SFunction "/3 -> loadShedding/1  "loadShedding"
  " SFunction "/4 -> bessReserveCal/1  "bessReserveCal"
  " Demux "/1 -> " Terminator "/1
  " SFunction "/1 -> " Demux "/1

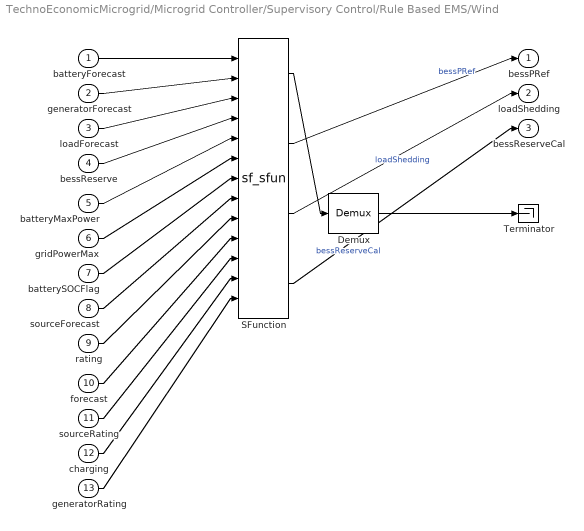
== system TechnoEconomicMicrogrid/Microgrid Controller/Supervisory Control/Rule Based EMS/Wind ==
  batteryForecast : Inport
  generatorForecast : Inport  Port=2
  loadForecast : Inport  Port=3
  bessReserve : Inport  Port=4
  batteryMaxPower : Inport  Port=5
  gridPowerMax : Inport  Port=6
  batterySOCFlag : Inport  Port=7
  sourceForecast : Inport  Port=8
  rating : Inport  Port=9
  forecast : Inport  Port=10
  sourceRating : Inport  Port=11
  charging : Inport  Port=12
  generatorRating : Inport  Port=13
  " Demux " : Demux  Outputs=1
  " SFunction " : S-Function  Tag=Stateflow S-Function 6  FunctionName=sf_sfun  PortCounts=[13 4]  SFunctionDeploymentMode=off  EnableBusSupport=off
  " Terminator " : Terminator
  bessPRef : Outport
  loadShedding : Outport  Port=2
  bessReserveCal : Outport  Port=3
  wires:
  batteryForecast/1 -> " SFunction "/1
  generatorForecast/1 -> " SFunction "/2
  loadForecast/1 -> " SFunction "/3
  bessReserve/1 -> " SFunction "/4
  batteryMaxPower/1 -> " SFunction "/5
  gridPowerMax/1 -> " SFunction "/6
  batterySOCFlag/1 -> " SFunction "/7
  sourceForecast/1 -> " SFunction "/8
  rating/1 -> " SFunction "/9
  forecast/1 -> " SFunction "/10
  sourceRating/1 -> " SFunction "/11
  charging/1 -> " SFunction "/12
  generatorRating/1 -> " SFunction "/13
  " SFunction "/2 -> bessPRef/1  "bessPRef"
  " SFunction "/3 -> loadShedding/1  "loadShedding"
  " SFunction "/4 -> bessReserveCal/1  "bessReserveCal"
  " Demux "/1 -> " Terminator "/1
  " SFunction "/1 -> " Demux "/1

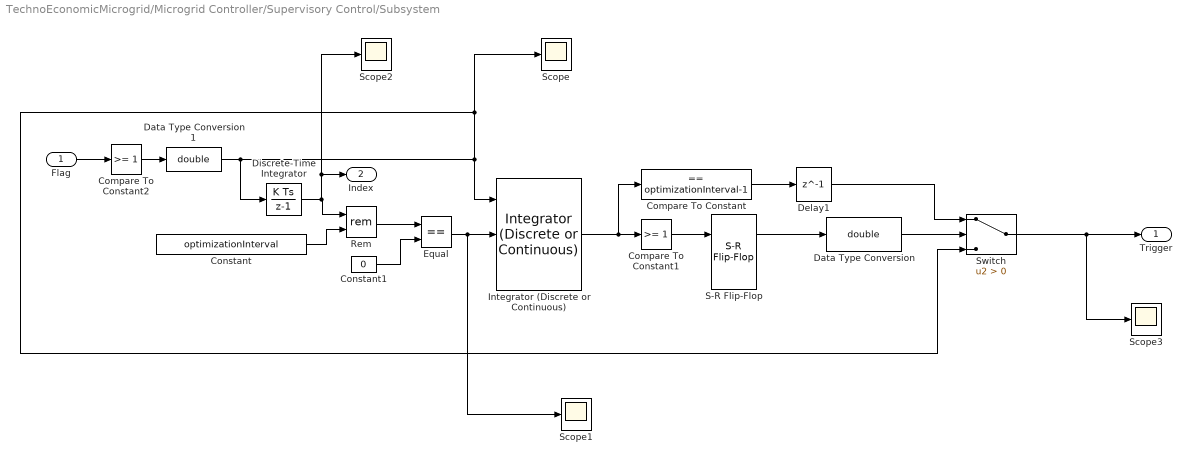
== system TechnoEconomicMicrogrid/Microgrid Controller/Supervisory Control/Subsystem ==
  Flag : Inport
  Compare To Constant : simulink/Logic and Bit Operations/Compare To Constant  relop===  const=optimizationInterval-1  OutDataTypeStr=boolean
  Compare To Constant1 : simulink/Logic and Bit Operations/Compare To Constant  relop=>=  const=1  OutDataTypeStr=boolean
  Compare To Constant2 : simulink/Logic and Bit Operations/Compare To Constant  relop=>=  const=1  OutDataTypeStr=boolean
  Constant : Constant  Value=optimizationInterval
  Constant1 : Constant  Value=0
  Data Type Conversion : DataTypeConversion  OutDataTypeStr=double  SaturateOnIntegerOverflow=off  RndMeth=Floor
  Data Type Conversion1 : DataTypeConversion  OutDataTypeStr=double  SaturateOnIntegerOverflow=off  RndMeth=Floor
  Delay1 : Delay  DelayLength=1
  Discrete-Time Integrator : DiscreteIntegrator  SampleTime=-1  ICPrevOutput=DiscIntNeverNeededParam  ICPrevScaledInput=DiscIntNeverNeededParam
  Equal : RelationalOperator  Operator===  OutDataTypeStr=boolean  RndMeth=Simplest  InputSameDT=off
  Integrator (Discrete or Continuous) : eeGeneralControl/Integrator (Discrete or Continuous)  LabelModeActiveChoice=Discrete  ExternalReset=rising  LimitType=Anti-windup  B=inf  A=-inf  Ts=-1
      settings: LibrarySourceBlock=|
      | ee_sl_lib/General Control/Integrator
      | (Discrete or Continuous)
  Rem : Math  Operator=rem
  S-R Flip-Flop : simulink_extras/Flip Flops/S-R Flip-Flop  initial_condition=0
  Scope{,1..3} (4 alike) : Scope
      Scope settings: ActiveDisplayYMinimum=-0.125  ActiveDisplayYMaximum=1.125  DataLoggingVariableName=ScopeData10
      Scope1 settings: ActiveDisplayYMinimum=-0.125  ActiveDisplayYMaximum=1.125  DataLoggingVariableName=ScopeData11
      Scope2 settings: ActiveDisplayYMinimum=-30  ActiveDisplayYMaximum=270  DataLoggingVariableName=ScopeData13
      Scope3 settings: ActiveDisplayYMinimum=-0.08025  ActiveDisplayYMaximum=1.0658  DataLoggingVariableName=ScopeData2
  Switch : Switch  Criteria=u2 > Threshold  SaturateOnIntegerOverflow=off  InputSameDT=off
  Trigger : Outport
  Index : Outport  Port=2
  wires:
  Flag/1 -> Compare To Constant2/1
  Constant/1 -> Rem/2
  Discrete-Time Integrator/1 -> Scope2/1, Index/1, Rem/1
  Compare To Constant1/1 -> S-R Flip-Flop/1
  Equal/1 -> Scope1/1, Integrator (Discrete or Continuous)/2
  Integrator (Discrete or Continuous)/1 -> Compare To Constant/1, Compare To Constant1/1
  Rem/1 -> Equal/1
  Constant1/1 -> Equal/2
  Data Type Conversion/1 -> Switch/2
  S-R Flip-Flop/1 -> Data Type Conversion/1
  Compare To Constant/1 -> Delay1/1
  Delay1/1 -> Switch/1
  Switch/1 -> Scope3/1, Trigger/1
  Compare To Constant2/1 -> Data Type Conversion1/1
  Data Type Conversion1/1 -> Discrete-Time Integrator/1, Scope/1, Switch/3, Integrator (Discrete or Continuous)/1

== stateflow chart TechnoEconomicMicrogrid/Microgrid Controller/Supervisory Control/Rule Based EMS/Solar ==
  (default) -> (junction 19) : % Battery Reference Generation
  (junction 62) -> (junction 83)
  (junction 19) -> (junction 62) [order 1] : [batterySOCFlag == true]
  (junction 83) -> (junction 85)
  (junction 19) -> (junction 18) [order 6]
  (junction 45) -> (junction 55) [order 3]
  (junction 19) -> (junction 20) [order 2] : [bessReserve > 0 && bessReserve > forecast*rating && bessPRef>=0]
  (junction 20) -> (junction 77) [order 2] : {bessPRef = batteryMaxPower;
      | bessReserveCal = batteryMaxPower;}
  (junction 19) -> (junction 45) [order 5] : [bessPRef < 0]
  (junction 19) -> (junction 21) [order 3] : [bessReserve > 0 && bessReserve < forecast*rating && bessPRef>=0]
  (junction 19) -> (junction 22) [order 4] : [forecast*rating <= 0 && bessPRef>=0 ]
  (junction 20) -> (junction 75) [order 1] : [forecast*rating+batteryForecast < batteryMaxPower]
  (junction 77) -> (junction 79)
  (junction 45) -> (junction 51) [order 2] : [forecast*rating >= 0 && forecast*rating < bessReserve]
  (junction 21) -> (junction 73)
  (junction 51) -> (junction 53) : {bessPRef = forecast*rating;
      | bessReserveCal = batteryMaxPower;}
  (junction 45) -> (junction 47) [order 1] : [forecast*rating > bessReserve]
  (junction 73) -> (junction 23) : {bessPRef = batteryMaxPower;
      | bessReserveCal = batteryMaxPower;
      | gridPower = loadForecast-bessPRef-sourceForecast*sourceRating-generatorForecast*generatorRating;
      | }
  (junction 75) -> (junction 28) : {bessPRef = forecast*rating+batteryForecast;
      | bessReserveCal = batteryMaxPower;}
  (junction 49) -> (junction 22)
  (junction 87) -> (junction 22)
  (junction 22) -> (junction 24) : {gridPower = loadForecast-sourceForecast*sourceRating-generatorForecast*generatorRating;}
  (junction 47) -> (junction 49) : {bessPRef = batteryMaxPower;
      | bessReserveCal = batteryMaxPower;}
  (junction 28) -> (junction 79)
  (junction 24) -> (junction 67) [order 2]
  (junction 23) -> (junction 67) [order 2]
  (junction 24) -> (junction 26) [order 1] : [gridPower > gridPowerMax]
  (junction 23) -> (junction 25) [order 1] : [gridPower > gridPowerMax]{excessLoad = gridPowerMax-gridPower;}
  (junction 26) -> (junction 29) : {loadShedding = true;}
  (junction 25) -> (junction 27) : {loadShedding = true;}
  (junction 85) -> (junction 87)
  data: batteryForecast input double; generatorForecast input double; loadForecast input double; bessPRef output double; bessReserve input double; batteryMaxPower input double; excessLoad data_store_memory; gridPowerMax input double; loadShedding output boolean; batterySOCFlag input boolean; sourceForecast input double; rating input double; forecast input double; sourceRating input double; gridPower local double; charging input; bessReserveCal output double; generatorRating input double

== matlab function TechnoEconomicMicrogrid/Microgrid Controller/Supervisory Control/Forecast ==
  data: battery input; wind input; solar input; generator input; batteryForecast output; windForecast output; solarForecast output; generatorForecast output; load input; time input; loadForecast output; normalizedWindPower input
function [batteryForecast,windForecast,solarForecast,generatorForecast,loadForecast] = fcn(battery,wind,solar,generator,load,time,normalizedWindPower)
    % Access the array in the base workspace

    % Get the specific element
    loadForecast = load(time+1);
    solarForecast = solar(time+1);
    windForecast = wind(time+1)*normalizedWindPower(time+1);
    generatorForecast = generator(time+1);
    batteryForecast = battery(time+1);
end

== stateflow chart TechnoEconomicMicrogrid/Microgrid Controller/Supervisory Control/Rule Based EMS ==
  state Start
  state Wind
  state Normal_Operation
    bessPRef = batteryForecast;
    loadShedding = false;
    state Discharging
      bessReserve = bessPRef-batteryMaxPower;
      discharging = true;
      charging = false;
    state Charging
      bessReserve = batteryMaxPower;
      charging = true;
      discharging = false;
    (default) -> Discharging [order 1] : [bessPRef > 0]
    (default) -> Charging [order 2]
    Discharging -> Charging : [batteryForecast < 0]
  state Solar
  (default) -> Start
  Start -> (junction 310) [order 1]
  Start -> (junction 316) [order 2] : [flag == 2]
  Start -> (junction 313) [order 3] : [flag == 1]
  Wind -> Wind [order 2] : [flag == 1]{bessReserve = bessReserveCal;}
  (junction 342) -> Wind
  (junction 340) -> (junction 342)
  Wind -> (junction 320) [order 1] : [flag == 0]
  (junction 313) -> Wind
  (junction 320) -> (junction 322)
  (junction 310) -> Normal_Operation : [flag == 0]
  (junction 316) -> (junction 345)
  Normal_Operation -> (junction 348) [order 2] : [flag == 2]
  Solar -> Solar [order 1] : [flag == 2]{bessReserve = batteryMaxPower - bessPRef;}
  (junction 345) -> Solar
  (junction 348) -> (junction 350)
  Normal_Operation -> (junction 336) [order 1]
  (junction 336) -> (junction 338) : [flag == 1]
  (junction 324) -> Normal_Operation
  (junction 332) -> Normal_Operation
  (junction 350) -> Solar
  Solar -> (junction 327) [order 2] : [flag == 0]
  (junction 327) -> (junction 330)
  (junction 330) -> (junction 332)
  (junction 322) -> (junction 324)
  (junction 338) -> (junction 340)
  data: bessReserve function_input; batteryMaxPower function_input; gridPowerMax function_input; rating function_input; sourceRating function_input; charging function_input; bessReserveCal function_output; generatorRating function_input; bessReserve function_input; batteryMaxPower function_input; gridPowerMax function_input; rating function_input; sourceRating function_input; charging function_input; bessReserveCal function_output; generatorRating function_input; batteryForecast input double; windForecast input double; solarForecast input; generatorForecast input double; loadForecast input double; bessPRef output double; excessLoad local double; loadShedding output boolean; batterySOCFlag input boolean; gridPowerMax parameter double; batteryMaxPower parameter double; windRating parameter double; bessReserve local double; gridPower local double; solarRating parameter; flag input; charging local boolean; discharging local boolean; bessReserveCal local double; generatorRating parameter double
